simulink model "OCT07_4_cs"  (Simulink 8.8)
settings: Solver=ode5  StartTime=0.0  StopTime=inf  FixedStep=1/20  RelTol=1e-3
model workspace (MAT data in the model file):
  mbox_table : struct (value not decoded)
  model_closed = 0
  sim_status = 0
PreLoadFcn:
  | check_NUTS_defined;
  | 
  | assignin('base',['model_closed_' bdroot],false);
InitFcn:
  | PreScanExperimentInitFcn(bdroot)
StopFcn:
  | PreScanExperimentStopFcn(bdroot)
undefined symbols (not defined in the file): DiscIntNeverNeededParam, InitImageOutputDir, lf, lr
libraries: PreScanSimulinkLibrary x4, PreScanUsefulBlocks x3
(part 1 of 2)
CloseFcn:
  | evalin('base',['clear model_closed_' bdroot]);
settings Model: Creator=PRESCAN  LastModifiedBy=yuntao891011
settings OptimizationCC: ExpressionDepthLimit=2147483647  InitFltsAndDblsToZero=on
settings DebuggingCC: SaveWithParameterizedLinksMsg=none  SignalResolutionControl=TryResolveAllWithWarning  MultiTaskDSMMsg=warning  MultiTaskCondExecSysMsg=none
settings GRTTargetCC: TargetFcnLib=ansi_tfl_tmw.mat

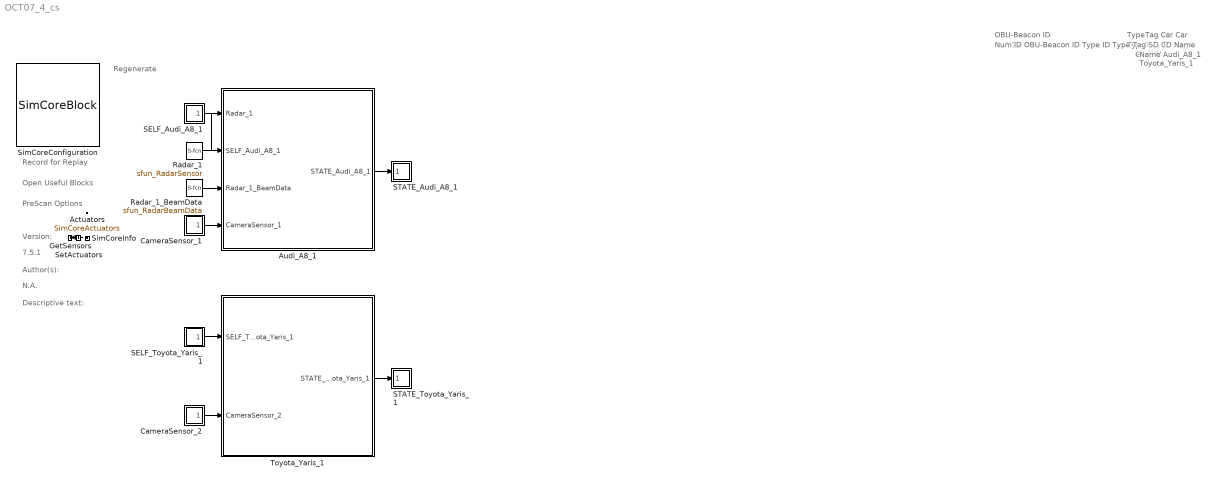
== system OCT07_4_cs ==
  note: Regenerate
  note: Record for Replay
  note: Open Useful Blocks
  note: PreScan Options
  note: Version:
  note: 7.5.1
  note: Author(s):
  note: N.A.
  note: Descriptive text:
  note: ID
      |
      | 2
      | 12
  note: OBU-Beacon ID
  note: TypeID
      |
      | 1
      | 1
  note: TypeTag
      |
      | Car
      | Car
  note: SD
      |
      | Y
      | Y
  note: CD
      |
      | N
      | N
  note: Name
      |
      | Audi_A8_1
      | Toyota_Yaris_1
  note: Num ID OBU-Beacon ID Type ID Type Tag SD CD Name
  Actuators : DataStoreMemory  DataStoreName=SimCoreActuators  InitialValue=zeros(30,1)  ShowAdditionalParam=off
  Audi_A8_1 : Subsystem  Tag=WorldObjectSubSystem  InitFcn=UniqueId = '14';
      mask Display: image(imread('Audi_A8.jpg'));color('white');text(0,0,' ID=2\n')
  CameraSensor_1 : Subsystem  Tag=CameraSensor  Priority=3  mask(PreScan Source Block: Camera Sensor){}
      mask help: The Camera Sensor provides a color or monochrome image.
      settings: DeleteFcn=PreScanBlockDeleteFcn;
      mask Help: eval('openHelp(457)')
      mask Display: image(imread('CameraSensor.png'))
  CameraSensor_2 : Subsystem  Tag=CameraSensor  Priority=3  mask(PreScan Source Block: Camera Sensor){}
      mask help: The Camera Sensor provides a color or monochrome image.
      settings: DeleteFcn=PreScanBlockDeleteFcn;
      mask Help: eval('openHelp(457)')
      mask Display: image(imread('CameraSensor.png'))
  GetSensors : Subsystem  Tag=GetSensors  Priority=2  mask(PreScan Simulation Core Block){NrOfSensors=16, TimeStep=1/20}
      mask prompts: NrOfSensors "Number of sensor values"; TimeStep "Timestep [s]"
      mask help:
      | Please do not remove this block from the PreScan compilation sheet,
      | as it contains essential configuration parameters for a PreScan simulation.
      settings: DeleteFcn=PreScanBlockDeleteFcn;
  Radar_1 : S-Function  Priority=3  LoadFcn=load('PrescanScannerSensorData.mat');load('PrescanScannerSensorMessage.mat')  FunctionName=sfun_RadarSensor  Parameters=timestepMask maxInputMessages maxOutputMessages sensorID detectableObjects  SFunctionDeploymentMode=off  EnableBusSupport=off  mask{timestepMask=1/20, maxInputMessages=0, maxOutputMessages=7, sensorID=15, detectableObjects=7}
      mask prompts: timestepMask "MATLAB timestep:"; maxInputMessages "Max input messages:"; maxOutputMessages "Max output messages:"; sensorID "Sensor ID:"; detectableObjects "Max detectable objects:"
      mask help: RadarSensor I/O
      mask Display: image(imread('Radar.png'))
  Radar_1_BeamData : S-Function  Priority=3  LoadFcn=load('PrescanScannerSensorBeamData.mat');load('PrescanScannerSensorBeamMessage.mat')  FunctionName=sfun_RadarBeamData  Parameters=timestepMask maxInputMessages maxOutputMessages sensorID detectableObjects  SFunctionDeploymentMode=off  EnableBusSupport=off  mask{timestepMask=1/20, maxInputMessages=0, maxOutputMessages=1, sensorID=15, detectableObjects=1}
      mask prompts: timestepMask "MATLAB timestep:"; maxInputMessages "Max input messages:"; maxOutputMessages "Max output messages:"; sensorID "Sensor ID:"; detectableObjects "Max detectable objects:"
      mask help: RadarSensor I/O
      mask Display: image(imread('BeamInfo.png'))
  SELF_Audi_A8_1 : Subsystem  Tag=SELF  Priority=3  mask(PreScan Source Block: SELF){PortName=SELF_Audi_A8_1, PortIndex=0, PortWidth=8, TimeStep=1/20}
      mask prompts: PortName "Auto-Assigned: Port Name [-]"; PortIndex "Auto-Assigned: Port Index [-]"; PortWidth "Auto-Assigned: Port Dimensions"; TimeStep "Auto-Assigned: Upload Period [s]"
      mask help:
      | The SELF port shows (state) information of the actor itself. The outputs are position in the experiment's axis system and the GPS coordinates, and the object's absolute velocity and compass heading.
      |
      | For more information, please click Help.
      settings: DeleteFcn=PreScanBlockDeleteFcn;
      mask Help: eval('openHelp(462)')
      mask Display: image(imread('GPS.png'))
  SELF_Toyota_Yaris_1 : Subsystem  Tag=SELF  Priority=3  mask(PreScan Source Block: SELF){PortName=SELF_Toyota_Yaris_1, PortIndex=8, PortWidth=8, TimeStep=1/20}
      mask prompts: PortName "Auto-Assigned: Port Name [-]"; PortIndex "Auto-Assigned: Port Index [-]"; PortWidth "Auto-Assigned: Port Dimensions"; TimeStep "Auto-Assigned: Upload Period [s]"
      mask help:
      | The SELF port shows (state) information of the actor itself. The outputs are position in the experiment's axis system and the GPS coordinates, and the object's absolute velocity and compass heading.
      |
      | For more information, please click Help.
      settings: DeleteFcn=PreScanBlockDeleteFcn;
      mask Help: eval('openHelp(462)')
      mask Display: image(imread('GPS.png'))
  STATE_Audi_A8_1 : Subsystem  Tag=State  Priority=0  mask(PreScan Sink Block: State){x0=0.70359420776367188, y0=-3.0454330444335937, z0=0.55, Roll0=0, Pitch0=0, Yaw0=0, TimeStep=1/20}
      mask prompts: x0 "Ini x-position VEHICLE wrt GLOBAL axis system [m]"; y0 "Ini y-position VEHICLE wrt GLOBAL axis system [m]"; z0 "Ini z-position VEHICLE wrt GLOBAL axis system [m]"; Roll0 "Ini roll-angle BODY wrt VEHICLE axis system [deg]"; Pitch0 "Ini pitch-angle BODY wrt VEHICLE axis system [deg]"; Yaw0 "Ini yaw-angle VEHICLE wrt GLOBAL axis system [deg]"; TimeStep "Time Step [s]"
      mask help:
      | The Actor State contains a vector signal of size (9x1), containing the following signals:
      |
      | -  Position                  (x,y,z)                                     [m]
      | -  Velocity                  (vx,vy,vz)                               [m/s]
      | -  Angles                    (Roll, Pitch, Yaw)                   [rad]
      |
      | The Actor state is defined in the global axis system.
      | The state is superponed on the Initial position defined in the GUI.
      |
      | For more information, please click Help.
      settings: DeleteFcn=PreScanBlockDeleteFcn;
      mask Help: eval('openHelp(222)')
      mask Display: image(imread('State.png'))
  STATE_Toyota_Yaris_1 : Subsystem  Tag=State  Priority=0  mask(PreScan Sink Block: State){x0=-12.185623168945313, y0=-3.0852584838867187, z0=0.57, Roll0=0, Pitch0=0, Yaw0=0, TimeStep=1/20}
      mask prompts: x0 "Ini x-position VEHICLE wrt GLOBAL axis system [m]"; y0 "Ini y-position VEHICLE wrt GLOBAL axis system [m]"; z0 "Ini z-position VEHICLE wrt GLOBAL axis system [m]"; Roll0 "Ini roll-angle BODY wrt VEHICLE axis system [deg]"; Pitch0 "Ini pitch-angle BODY wrt VEHICLE axis system [deg]"; Yaw0 "Ini yaw-angle VEHICLE wrt GLOBAL axis system [deg]"; TimeStep "Time Step [s]"
      mask help:
      | The Actor State contains a vector signal of size (9x1), containing the following signals:
      |
      | -  Position                  (x,y,z)                                     [m]
      | -  Velocity                  (vx,vy,vz)                               [m/s]
      | -  Angles                    (Roll, Pitch, Yaw)                   [rad]
      |
      | The Actor state is defined in the global axis system.
      | The state is superponed on the Initial position defined in the GUI.
      |
      | For more information, please click Help.
      settings: DeleteFcn=PreScanBlockDeleteFcn;
      mask Help: eval('openHelp(222)')
      mask Display: image(imread('State.png'))
  SetActuators : Subsystem  Tag=SetActuators  Priority=1  mask(PreScan Simulation Core Block){TimeStep=1/20, NrOfActuators=30}
      mask prompts: TimeStep "Timestep [s]"; NrOfActuators "Number of actuator values"
      mask help:
      | Please do not remove this block from the PreScan compilation sheet,
      | as it contains essential configuration parameters for a PreScan simulation.
      settings: DeleteFcn=PreScanBlockDeleteFcn;
  SimCoreConfiguration : M-S-Function  Tag=SimCoreConfiguration  Description=AFF8662A0A05274BB8B75CAA8617EE4EF722880921021BB04CFBF9D9D8032257  FunctionName=SimCoreBlock  Parameters=ExperimentXML PortsXML SimulationCore HostName CheckStart EnableLog RfR EnableGPUAccel ShowComputationTime  mask(PreScan Simulation Core Configurator){SimulationCore=NUTS, HostName=0, CheckStart=0, prescanversion='7.5.1', EnableLog=off, RfR=0, EnableGPUAccel=off, ShowComputationTime=off}
      mask prompts: SimulationCore "Simulation Core"; HostName "Simulation Host"; CheckStart "Show START Dialog"; prescanversion "PreScan Version"; EnableLog "Create TA Log"; RfR "Record for Replay"; EnableGPUAccel "Enable GPU Acceleration"; ShowComputationTime "Show ComputationTime Scope"
      mask help:
      | Please do not remove this block from the PreScan compilation sheet,
      | as it contains essential configuration parameter for a PreScan simulation.
      mask init:
      | model = bdroot;
      | ExperimentXML = [model(1:end-3) '.pex'];
      | PortsXML = [model '_ports.pcd'];
      settings: DeleteFcn=PreScanBlockDeleteFcn;  ModelCloseFcn=assignin('base',['model_closed_' bdroot],true);
      mask Help: eval('openHelp(812)')
      mask Display: image(imread('prescanlogo.ico'))
  SimCoreInfo : Subsystem  Tag=SimCoreInfo
  Toyota_Yaris_1 : Subsystem  Tag=WorldObjectSubSystem  InitFcn=UniqueId = '28';
      mask Display: image(imread('Toyota_Yaris.jpg'));color('white');text(0,0,' ID=12\n')
  wires:
  SetActuators/1(dummy) -> GetSensors/1(dummy)
  Audi_A8_1/1(STATE_Audi_A8_1) -> STATE_Audi_A8_1/1(State)
  SELF_Audi_A8_1/1(U) -> Audi_A8_1/2(SELF_Audi_A8_1)
  Radar_1/1 -> Audi_A8_1/1(Radar_1)
  Radar_1_BeamData/1 -> Audi_A8_1/3(Radar_1_BeamData)
  CameraSensor_1/1(U1) -> Audi_A8_1/4(CameraSensor_1)
  Toyota_Yaris_1/1(STATE_Toyota_Yaris_1) -> STATE_Toyota_Yaris_1/1(State)
  SELF_Toyota_Yaris_1/1(U) -> Toyota_Yaris_1/1(SELF_Toyota_Yaris_1)
  CameraSensor_2/1(U1) -> Toyota_Yaris_1/2(CameraSensor_2)

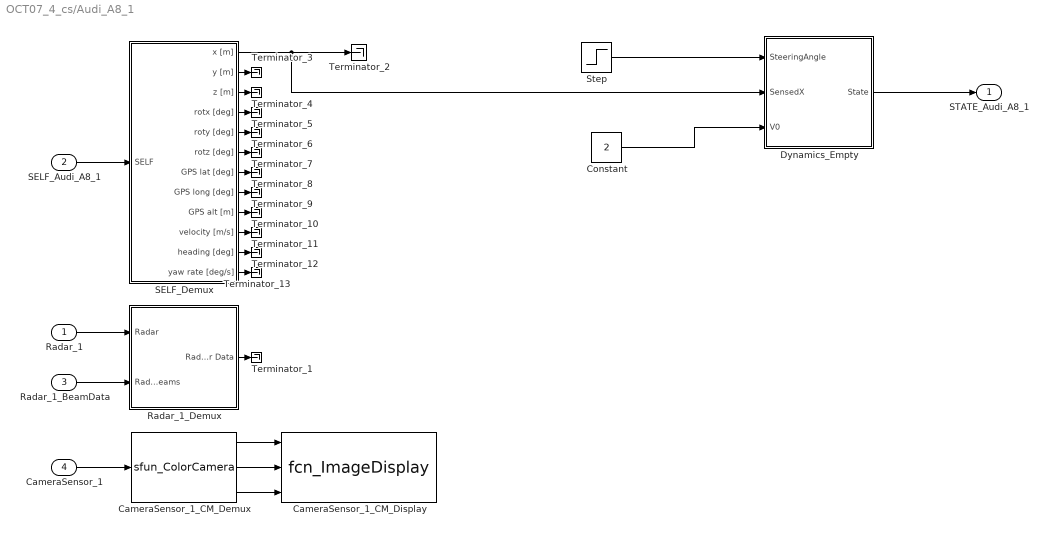
== system OCT07_4_cs/Audi_A8_1 ==
  Radar_1 : Inport  Tag=RadarInport  OutDataTypeStr=Bus: PRESCAN_SCANNERSENSORMESSAGE
  SELF_Audi_A8_1 : Inport  Tag=SELFInport  Port=2
  Radar_1_BeamData : Inport  Tag=RadarInport  Port=3  OutDataTypeStr=Bus: PRESCAN_SCANNERSENSORBEAMMESSAGE
  CameraSensor_1 : Inport  Tag=CameraSensorInport  Port=4  SampleTime=1/20
  CameraSensor_1_CM_Demux : S-Function  Tag=CameraSensor_Color_Demux  FunctionName=sfun_ColorCamera  Parameters=[VerticalResolution HorizontalResolution] FrameRate SensorName CameraType SharedMemTag SharedMemRightTag DataType  SFunctionDeploymentMode=off  EnableBusSupport=off  mask{HorizontalResolution=320, VerticalResolution=240, FrameRate=20, SensorName=CameraSensor_1, CameraType=Mono, SharedMemTag=CameraSensor_1_monoBeam_viewer_RGB, SharedMemRightTag=CameraSensor_1_StereoRight_viewer_RGB, DataType=uint8}
      mask prompts: HorizontalResolution "User Specified: Horizontal Resolution [pixels]"; VerticalResolution "User Specified: Vertical Resolution [pixels]"; FrameRate "User Specified: Frame Rate [Hz]"; SensorName "User Specified: Camera Sensor Name"; CameraType "Camera Type"; SharedMemTag "Tag for shared memory for main img"; SharedMemRightTag "Tag for shared memory for right img"; DataType "Image Data Type"
      mask init:
      | if CameraType==1
      |     CameraTypeName='MONO';
      |     PortNumber=0;
      | else
      |     CameraTypeName='STEREO';
      |     PortNumber=3;
      | end
      settings: DeleteFcn=PreScanBlockDeleteFcn;
      mask TypeOptions CameraType: Mono | Stereo
      mask TypeOptions DataType: uint8 | single
      mask Display:
      | fprintf('%s CAMERA:\n Color\n %s \n V: %d x %d \n %d fps',CameraTypeName,SensorName,VerticalResolution,HorizontalResolution,FrameRate)
      | port_label('output',1,'R')
      | port_label('output',2,'G')
      | port_label('output',3,'B')
      | port_label('output',PortNumber+1,'R')
      | port_label('output',PortNumber+2,'G')
      | port_label('output',PortNumber+3,'B')
  CameraSensor_1_CM_Display : M-S-Function  Tag=CameraSensor_Color_Display  InitFcn=InitImageOutputDir(gcb);  FunctionName=fcn_ImageDisplay  Parameters=SensorName EnableDisplay EnablePosition DisplayPosition FigureHandle SaveResults BitmapFormat TempOutputDir CameraType DataType  mask(PreScan Color Display Block){SensorName=CameraSensor_1, EnableDisplay=on, EnablePosition=off, DisplayPosition=[10 10 320 240], FigureHandle=200, SaveResults=off, Format=PNG, TempOutputDir=0, CameraType=Mono, DataType=uint8}
      mask prompts: SensorName "User Specified: Title of Display"; EnableDisplay "Active"; EnablePosition "Set Display window position"; DisplayPosition "Display window position [xpos ypos width height]"; FigureHandle "Unique Handle"; SaveResults "Save results"; TempOutputDir "OutputDir"; CameraType "Camera Type"; DataType "Image Data Type"
      mask help: This block displays the RGB output of a PreScan camera sensor.
      mask init:
      | if EnableDisplay
      |     EnableString='';
      |     EnableColor='gray';
      | else
      |     EnableString='INACTIVE';
      |     EnableColor='red';
      | end
      | switch Format
      |     case 1
      |         BitmapFormat = 'png';
      |     case 2
      |         BitmapFormat = 'bmp';
      |     case 3
      |         BitmapFormat = 'jpg';
      | end 
      | if CameraType==1
      |     CameraTypeName='MONO';
      |     PortNumber=0;
      | else
      |     CameraTypeName='STEREO';
      |     PortNumber=3;
      | end
      settings: CopyFcn=CopyFcnDisplay  DeleteFcn=PreScanBlockDeleteFcn;  ModelCloseFcn=fcn_ImageDisplay_ModelCloseFcn
      mask Help: eval('openHelp(457)')
      mask Callback EnablePosition:
      | MV=get_param(gcb,'MaskVisibilities');
      | if strcmp(get_param(gcb,'EnablePosition'),'on')
      |     MV{4}='on';
      | else
      |     MV{4}='off';
      | end
      | set_param(gcb,'MaskVisibilities',MV);
      mask TypeOptions Format: PNG | BMP | JPG
      mask TypeOptions CameraType: Mono | Stereo
      mask TypeOptions DataType: uint8 | single
      mask Display:
      | color(EnableColor);
      | fprintf('%s\n DISPLAY:\n Color \n %s',EnableString,SensorName)
      | port_label('input',1,'R')
      | port_label('input',2,'G')
      | port_label('input',3,'B')
      | port_label('input',PortNumber+1,'R')
      | port_label('input',PortNumber+2,'G')
      | port_label('input',PortNumber+3,'B')
  Constant : Constant  Value=2
  Dynamics_Empty : Subsystem  Tag=Dynamics_Empty
  Radar_1_Demux : Subsystem  TreatAsAtomicUnit=on  mask(PreScan Demux Block: Radar){MAXMESSAGES=7}
      mask prompts: MAXMESSAGES "Number of Objects"
      mask help:
      | The Radar Sensor is a detailed sensor based on a physical radar
      | model that includes Antenna GAIN Maps (AGM) and atmospheric
      | attenuation.
      |
      | For more information, please click Help.
      mask Help: eval('openHelp(431)')
      mask Display:
      | port_label('input',1,'Radar')
      | port_label('output',1,'Radar Data')
  SELF_Demux : Subsystem  Tag=DemuxSELF  mask(PreScan Demux Block:){}
      settings: DeleteFcn=PreScanBlockDeleteFcn;
      mask Display:
      | port_label('output',1,'x [m]')
      | port_label('output',2,'y [m]')
      | port_label('output',3,'z [m]','texmode','on')
      | port_label('output',4,'Rotx [deg]','texmode','on')
      | port_label('output',5,'Roty [deg]','texmode','on')
      | port_label('output',6,'Rotz [deg]','texmode','on')
      | port_label('output',7,'GPS lat [deg]','texmode','on')
      | port_label('output',8,'GPS long [deg]','texmode','on')
      | port_label('output',9,'GPS alt [m]','texmode','on')
      | port_label('output',10,'Velocity [m/s]')
      | port_label('output',11,'Heading [deg]')
      | port_label('output',12,'Yaw rate [deg/s]')
  Step : Step  Time=0  After=10  SampleTime=0
  Terminator_{1..13} (13 alike) : Terminator
  STATE_Audi_A8_1 : Outport  Tag=StateOutport
  wires:
  Step/1 -> Dynamics_Empty/1(SteeringAngle)
  Constant/1 -> Dynamics_Empty/3(V0)
  SELF_Audi_A8_1/1 -> SELF_Demux/1(SELF)
  Radar_1/1 -> Radar_1_Demux/1(Radar)
  Radar_1_BeamData/1 -> Radar_1_Demux/2(RadarBeams)
  CameraSensor_1_CM_Demux/1 -> CameraSensor_1_CM_Display/1
  CameraSensor_1_CM_Demux/2 -> CameraSensor_1_CM_Display/2
  CameraSensor_1_CM_Demux/3 -> CameraSensor_1_CM_Display/3
  CameraSensor_1/1 -> CameraSensor_1_CM_Demux/1
  Dynamics_Empty/1(State) -> STATE_Audi_A8_1/1
  Radar_1_Demux/1(Radar Data) -> Terminator_1/1
  SELF_Demux/1(x [m]) -> Dynamics_Empty/2("SensedX "), Terminator_2/1
  SELF_Demux/2(y [m]) -> Terminator_3/1
  SELF_Demux/3(z [m]) -> Terminator_4/1
  SELF_Demux/4(rotx [deg]) -> Terminator_5/1
  SELF_Demux/5(roty [deg]) -> Terminator_6/1
  SELF_Demux/6(rotz [deg]) -> Terminator_7/1
  SELF_Demux/7(GPS lat [deg]) -> Terminator_8/1
  SELF_Demux/8(GPS long [deg]) -> Terminator_9/1
  SELF_Demux/9(GPS alt [m]) -> Terminator_10/1
  SELF_Demux/10(velocity [m/s]) -> Terminator_11/1
  SELF_Demux/11(heading [deg]) -> Terminator_12/1
  SELF_Demux/12(yaw rate [deg/s]) -> Terminator_13/1

== system OCT07_4_cs/CameraSensor_1 ==
  Demux : Demux  Outputs=[1 -1]
  Terminator : Terminator
  U1 : Outport
  wires:
  Demux/2 -> Terminator/1
  Demux/1 -> U1/1
  [SimCoreSensors] -> Demux/1

== system OCT07_4_cs/CameraSensor_2 ==
  Demux : Demux  Outputs=[1 -1]
  Terminator : Terminator
  U1 : Outport
  wires:
  Demux/2 -> Terminator/1
  Demux/1 -> U1/1
  [SimCoreSensors] -> Demux/1

== system OCT07_4_cs/GetSensors ==
  dummy : Inport
  GetSensors : M-S-Function  FunctionName=GetSensorsBlock  Parameters=TimeStep NrOfSensors
  tag scope: SimCoreSensors=global
  wires:
  GetSensors/1 -> [SimCoreSensors]
  dummy/1 -> GetSensors/1

== system OCT07_4_cs/SELF_Audi_A8_1 ==
  Selector : Selector  IndexMode=Zero-based  IndexOptions=Starting index (dialog)  Indices=PortIndex  OutputSizes=PortWidth(1)
  U : Outport
  wires:
  Selector/1 -> U/1
  [SimCoreSensors] -> Selector/1

== system OCT07_4_cs/SELF_Toyota_Yaris_1 ==
  Selector : Selector  IndexMode=Zero-based  IndexOptions=Starting index (dialog)  Indices=PortIndex  OutputSizes=PortWidth(1)
  U : Outport
  wires:
  Selector/1 -> U/1
  [SimCoreSensors] -> Selector/1

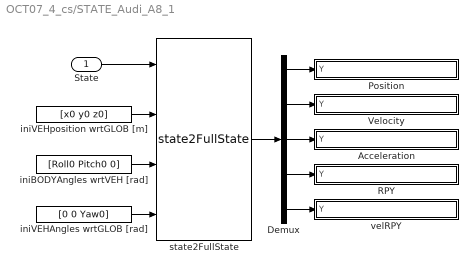
== system OCT07_4_cs/STATE_Audi_A8_1 ==
  State : Inport  SampleTime=TimeStep
  Acceleration : Subsystem  mask(ToSensorWorld){PortName=Acceleration_Audi_A8_1, PortIndex=6, PortWidth=3, TimeStep=1/20}
      mask prompts: PortName "Port Name [-]"; PortIndex "Index [-]"; PortWidth "Port Dimensions [-]"; TimeStep "Upload Period [s]"
      mask help: Sends signal(s) from Simulink to the Sensor World
      mask Help:
      | Sends signal(s) from Simulink to the Sensor World.
      | 
      | - Port Name [-]: specifies the name of the output terminal of the Simulink block.
      | - Index [-]: specifies the start position in the output vector sent to the Sensor World
      | - Port dimensions [-]: specifies the width (number of scalars) of the output port
      | - Upload period [s]: specifies the upload period (in seconds) of the port.
      mask Display: port_label('input', 1, PortName)
  Demux : Demux  Outputs=5
  Position : Subsystem  mask(ToSensorWorld){PortName=Position_Audi_A8_1, PortIndex=0, PortWidth=3, TimeStep=1/20}
      mask prompts: PortName "Port Name [-]"; PortIndex "Index [-]"; PortWidth "Port Dimensions [-]"; TimeStep "Upload Period [s]"
      mask help: Sends signal(s) from Simulink to the Sensor World
      mask Help:
      | Sends signal(s) from Simulink to the Sensor World.
      | 
      | - Port Name [-]: specifies the name of the output terminal of the Simulink block.
      | - Index [-]: specifies the start position in the output vector sent to the Sensor World
      | - Port dimensions [-]: specifies the width (number of scalars) of the output port
      | - Upload period [s]: specifies the upload period (in seconds) of the port.
      mask Display: port_label('input', 1, PortName)
  RPY : Subsystem  mask(ToSensorWorld){PortName=RPY_Audi_A8_1, PortIndex=9, PortWidth=3, TimeStep=1/20}
      mask prompts: PortName "Port Name [-]"; PortIndex "Index [-]"; PortWidth "Port Dimensions [-]"; TimeStep "Upload Period [s]"
      mask help: Sends signal(s) from Simulink to the Sensor World
      mask Help:
      | Sends signal(s) from Simulink to the Sensor World.
      | 
      | - Port Name [-]: specifies the name of the output terminal of the Simulink block.
      | - Index [-]: specifies the start position in the output vector sent to the Sensor World
      | - Port dimensions [-]: specifies the width (number of scalars) of the output port
      | - Upload period [s]: specifies the upload period (in seconds) of the port.
      mask Display: port_label('input', 1, PortName)
  Velocity : Subsystem  mask(ToSensorWorld){PortName=Velocity_Audi_A8_1, PortIndex=3, PortWidth=3, TimeStep=1/20}
      mask prompts: PortName "Port Name [-]"; PortIndex "Index [-]"; PortWidth "Port Dimensions [-]"; TimeStep "Upload Period [s]"
      mask help: Sends signal(s) from Simulink to the Sensor World
      mask Help:
      | Sends signal(s) from Simulink to the Sensor World.
      | 
      | - Port Name [-]: specifies the name of the output terminal of the Simulink block.
      | - Index [-]: specifies the start position in the output vector sent to the Sensor World
      | - Port dimensions [-]: specifies the width (number of scalars) of the output port
      | - Upload period [s]: specifies the upload period (in seconds) of the port.
      mask Display: port_label('input', 1, PortName)
  iniBODYAngles wrtVEH [rad] : Constant  Value=[Roll0 Pitch0 0]  SampleTime=TimeStep
  iniVEHAngles wrtGLOB [rad] : Constant  Value=[0 0 Yaw0]  SampleTime=TimeStep
  iniVEHposition wrtGLOB [m] : Constant  Value=[x0 y0 z0]  SampleTime=TimeStep
  state2FullState : PreScanSimulinkLibrary/state2FullState  SystemSampleTime=-1
  velRPY : Subsystem  mask(ToSensorWorld){PortName=velRPY_Audi_A8_1, PortIndex=12, PortWidth=3, TimeStep=1/20}
      mask prompts: PortName "Port Name [-]"; PortIndex "Index [-]"; PortWidth "Port Dimensions [-]"; TimeStep "Upload Period [s]"
      mask help: Sends signal(s) from Simulink to the Sensor World
      mask Help:
      | Sends signal(s) from Simulink to the Sensor World.
      | 
      | - Port Name [-]: specifies the name of the output terminal of the Simulink block.
      | - Index [-]: specifies the start position in the output vector sent to the Sensor World
      | - Port dimensions [-]: specifies the width (number of scalars) of the output port
      | - Upload period [s]: specifies the upload period (in seconds) of the port.
      mask Display: port_label('input', 1, PortName)
  wires:
  Demux/5 -> velRPY/1(Y)
  Demux/4 -> RPY/1(Y)
  Demux/3 -> Acceleration/1(Y)
  Demux/2 -> Velocity/1(Y)
  Demux/1 -> Position/1(Y)
  State/1 -> state2FullState/1
  state2FullState/1 -> Demux/1
  iniVEHposition wrtGLOB [m]/1 -> state2FullState/2
  iniBODYAngles wrtVEH [rad]/1 -> state2FullState/3
  iniVEHAngles wrtGLOB [rad]/1 -> state2FullState/4

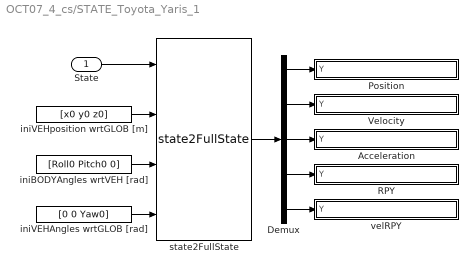
== system OCT07_4_cs/STATE_Toyota_Yaris_1 ==
  State : Inport  SampleTime=TimeStep
  Acceleration : Subsystem  mask(ToSensorWorld){PortName=Acceleration_Toyota_Yaris_1, PortIndex=21, PortWidth=3, TimeStep=1/20}
      mask prompts: PortName "Port Name [-]"; PortIndex "Index [-]"; PortWidth "Port Dimensions [-]"; TimeStep "Upload Period [s]"
      mask help: Sends signal(s) from Simulink to the Sensor World
      mask Help:
      | Sends signal(s) from Simulink to the Sensor World.
      | 
      | - Port Name [-]: specifies the name of the output terminal of the Simulink block.
      | - Index [-]: specifies the start position in the output vector sent to the Sensor World
      | - Port dimensions [-]: specifies the width (number of scalars) of the output port
      | - Upload period [s]: specifies the upload period (in seconds) of the port.
      mask Display: port_label('input', 1, PortName)
  Demux : Demux  Outputs=5
  Position : Subsystem  mask(ToSensorWorld){PortName=Position_Toyota_Yaris_1, PortIndex=15, PortWidth=3, TimeStep=1/20}
      mask prompts: PortName "Port Name [-]"; PortIndex "Index [-]"; PortWidth "Port Dimensions [-]"; TimeStep "Upload Period [s]"
      mask help: Sends signal(s) from Simulink to the Sensor World
      mask Help:
      | Sends signal(s) from Simulink to the Sensor World.
      | 
      | - Port Name [-]: specifies the name of the output terminal of the Simulink block.
      | - Index [-]: specifies the start position in the output vector sent to the Sensor World
      | - Port dimensions [-]: specifies the width (number of scalars) of the output port
      | - Upload period [s]: specifies the upload period (in seconds) of the port.
      mask Display: port_label('input', 1, PortName)
  RPY : Subsystem  mask(ToSensorWorld){PortName=RPY_Toyota_Yaris_1, PortIndex=24, PortWidth=3, TimeStep=1/20}
      mask prompts: PortName "Port Name [-]"; PortIndex "Index [-]"; PortWidth "Port Dimensions [-]"; TimeStep "Upload Period [s]"
      mask help: Sends signal(s) from Simulink to the Sensor World
      mask Help:
      | Sends signal(s) from Simulink to the Sensor World.
      | 
      | - Port Name [-]: specifies the name of the output terminal of the Simulink block.
      | - Index [-]: specifies the start position in the output vector sent to the Sensor World
      | - Port dimensions [-]: specifies the width (number of scalars) of the output port
      | - Upload period [s]: specifies the upload period (in seconds) of the port.
      mask Display: port_label('input', 1, PortName)
  Velocity : Subsystem  mask(ToSensorWorld){PortName=Velocity_Toyota_Yaris_1, PortIndex=18, PortWidth=3, TimeStep=1/20}
      mask prompts: PortName "Port Name [-]"; PortIndex "Index [-]"; PortWidth "Port Dimensions [-]"; TimeStep "Upload Period [s]"
      mask help: Sends signal(s) from Simulink to the Sensor World
      mask Help:
      | Sends signal(s) from Simulink to the Sensor World.
      | 
      | - Port Name [-]: specifies the name of the output terminal of the Simulink block.
      | - Index [-]: specifies the start position in the output vector sent to the Sensor World
      | - Port dimensions [-]: specifies the width (number of scalars) of the output port
      | - Upload period [s]: specifies the upload period (in seconds) of the port.
      mask Display: port_label('input', 1, PortName)
  iniBODYAngles wrtVEH [rad] : Constant  Value=[Roll0 Pitch0 0]  SampleTime=TimeStep
  iniVEHAngles wrtGLOB [rad] : Constant  Value=[0 0 Yaw0]  SampleTime=TimeStep
  iniVEHposition wrtGLOB [m] : Constant  Value=[x0 y0 z0]  SampleTime=TimeStep
  state2FullState : PreScanSimulinkLibrary/state2FullState  SystemSampleTime=-1
  velRPY : Subsystem  mask(ToSensorWorld){PortName=velRPY_Toyota_Yaris_1, PortIndex=27, PortWidth=3, TimeStep=1/20}
      mask prompts: PortName "Port Name [-]"; PortIndex "Index [-]"; PortWidth "Port Dimensions [-]"; TimeStep "Upload Period [s]"
      mask help: Sends signal(s) from Simulink to the Sensor World
      mask Help:
      | Sends signal(s) from Simulink to the Sensor World.
      | 
      | - Port Name [-]: specifies the name of the output terminal of the Simulink block.
      | - Index [-]: specifies the start position in the output vector sent to the Sensor World
      | - Port dimensions [-]: specifies the width (number of scalars) of the output port
      | - Upload period [s]: specifies the upload period (in seconds) of the port.
      mask Display: port_label('input', 1, PortName)
  wires:
  Demux/5 -> velRPY/1(Y)
  Demux/4 -> RPY/1(Y)
  Demux/3 -> Acceleration/1(Y)
  Demux/2 -> Velocity/1(Y)
  Demux/1 -> Position/1(Y)
  State/1 -> state2FullState/1
  state2FullState/1 -> Demux/1
  iniVEHposition wrtGLOB [m]/1 -> state2FullState/2
  iniBODYAngles wrtVEH [rad]/1 -> state2FullState/3
  iniVEHAngles wrtGLOB [rad]/1 -> state2FullState/4

== system OCT07_4_cs/SetActuators ==
  Bus Creator : BusCreator  Inputs=1
  Data Store Read : DataStoreRead  DataStoreName=SimCoreActuators  SampleTime=TimeStep
  SendActuators : M-S-Function  FunctionName=SendActuatorsBlock  Parameters=TimeStep NrOfActuators
  dummy : Outport
  tag scope: SimCoreInfo=global
  wires:
  Bus Creator/1 -> [SimCoreInfo]  "SimCore"
  SendActuators/2 -> Bus Creator/1  "ComputationTime[s]"
  SendActuators/1 -> dummy/1
  Data Store Read/1 -> SendActuators/1

== system OCT07_4_cs/SimCoreInfo ==
  Bus Selector : BusSelector  OutputSignals=ComputationTime[s]
  Time : Scope
  wires:
  Bus Selector/1 -> Time/1  "<ComputationTime[s]>"
  [SimCoreInfo] -> Bus Selector/1

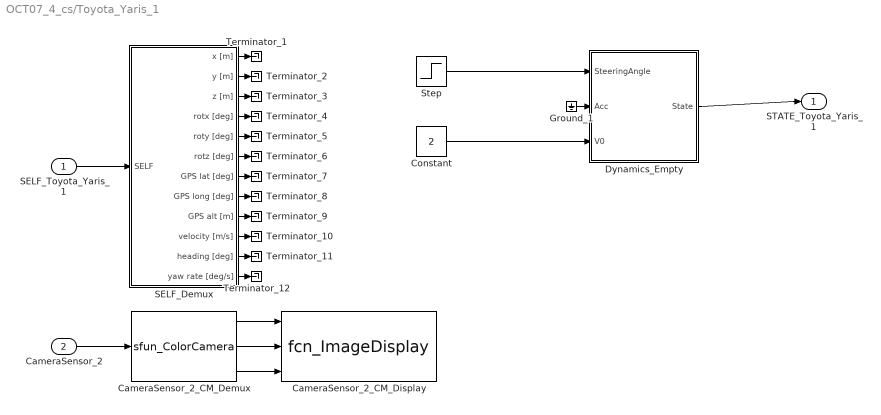
== system OCT07_4_cs/Toyota_Yaris_1 ==
  SELF_Toyota_Yaris_1 : Inport  Tag=SELFInport
  CameraSensor_2 : Inport  Tag=CameraSensorInport  Port=2  SampleTime=1/20
  CameraSensor_2_CM_Demux : S-Function  Tag=CameraSensor_Color_Demux  FunctionName=sfun_ColorCamera  Parameters=[VerticalResolution HorizontalResolution] FrameRate SensorName CameraType SharedMemTag SharedMemRightTag DataType  SFunctionDeploymentMode=off  EnableBusSupport=off  mask{HorizontalResolution=500, VerticalResolution=375, FrameRate=20, SensorName=CameraSensor_2, CameraType=Mono, SharedMemTag=CameraSensor_2_monoBeam_viewer_RGB, SharedMemRightTag=CameraSensor_2_StereoRight_viewer_RGB, DataType=uint8}
      mask prompts: HorizontalResolution "User Specified: Horizontal Resolution [pixels]"; VerticalResolution "User Specified: Vertical Resolution [pixels]"; FrameRate "User Specified: Frame Rate [Hz]"; SensorName "User Specified: Camera Sensor Name"; CameraType "Camera Type"; SharedMemTag "Tag for shared memory for main img"; SharedMemRightTag "Tag for shared memory for right img"; DataType "Image Data Type"
      mask init:
      | if CameraType==1
      |     CameraTypeName='MONO';
      |     PortNumber=0;
      | else
      |     CameraTypeName='STEREO';
      |     PortNumber=3;
      | end
      settings: DeleteFcn=PreScanBlockDeleteFcn;
      mask TypeOptions CameraType: Mono | Stereo
      mask TypeOptions DataType: uint8 | single
      mask Display:
      | fprintf('%s CAMERA:\n Color\n %s \n V: %d x %d \n %d fps',CameraTypeName,SensorName,VerticalResolution,HorizontalResolution,FrameRate)
      | port_label('output',1,'R')
      | port_label('output',2,'G')
      | port_label('output',3,'B')
      | port_label('output',PortNumber+1,'R')
      | port_label('output',PortNumber+2,'G')
      | port_label('output',PortNumber+3,'B')
  CameraSensor_2_CM_Display : M-S-Function  Tag=CameraSensor_Color_Display  InitFcn=InitImageOutputDir(gcb);  FunctionName=fcn_ImageDisplay  Parameters=SensorName EnableDisplay EnablePosition DisplayPosition FigureHandle SaveResults BitmapFormat TempOutputDir CameraType DataType  mask(PreScan Color Display Block){SensorName=CameraSensor_2, EnableDisplay=on, EnablePosition=off, DisplayPosition=[10 10 500 375], FigureHandle=1200, SaveResults=off, Format=PNG, TempOutputDir=0, CameraType=Mono, DataType=uint8}
      mask prompts: SensorName "User Specified: Title of Display"; EnableDisplay "Active"; EnablePosition "Set Display window position"; DisplayPosition "Display window position [xpos ypos width height]"; FigureHandle "Unique Handle"; SaveResults "Save results"; TempOutputDir "OutputDir"; CameraType "Camera Type"; DataType "Image Data Type"
      mask help: This block displays the RGB output of a PreScan camera sensor.
      mask init: same as OCT07_4_cs/Audi_A8_1/CameraSensor_1_CM_Display
      settings: CopyFcn=CopyFcnDisplay  DeleteFcn=PreScanBlockDeleteFcn;  ModelCloseFcn=fcn_ImageDisplay_ModelCloseFcn
      mask Help: eval('openHelp(457)')
      mask Callback EnablePosition:
      | MV=get_param(gcb,'MaskVisibilities');
      | if strcmp(get_param(gcb,'EnablePosition'),'on')
      |     MV{4}='on';
      | else
      |     MV{4}='off';
      | end
      | set_param(gcb,'MaskVisibilities',MV);
      mask TypeOptions Format: PNG | BMP | JPG
      mask TypeOptions CameraType: Mono | Stereo
      mask TypeOptions DataType: uint8 | single
      mask Display:
      | color(EnableColor);
      | fprintf('%s\n DISPLAY:\n Color \n %s',EnableString,SensorName)
      | port_label('input',1,'R')
      | port_label('input',2,'G')
      | port_label('input',3,'B')
      | port_label('input',PortNumber+1,'R')
      | port_label('input',PortNumber+2,'G')
      | port_label('input',PortNumber+3,'B')
  Constant : Constant  Value=2
  Dynamics_Empty : Subsystem  Tag=Dynamics_Empty
      mask Display: port_label('output', 1, 'State');text(0,0,' Empty\n')
  Ground_1 : Ground
  SELF_Demux : Subsystem  Tag=DemuxSELF  mask(PreScan Demux Block:){}
      settings: DeleteFcn=PreScanBlockDeleteFcn;
      mask Display:
      | port_label('output',1,'x [m]')
      | port_label('output',2,'y [m]')
      | port_label('output',3,'z [m]','texmode','on')
      | port_label('output',4,'Rotx [deg]','texmode','on')
      | port_label('output',5,'Roty [deg]','texmode','on')
      | port_label('output',6,'Rotz [deg]','texmode','on')
      | port_label('output',7,'GPS lat [deg]','texmode','on')
      | port_label('output',8,'GPS long [deg]','texmode','on')
      | port_label('output',9,'GPS alt [m]','texmode','on')
      | port_label('output',10,'Velocity [m/s]')
      | port_label('output',11,'Heading [deg]')
      | port_label('output',12,'Yaw rate [deg/s]')
  Step : Step  Time=0  After=10  SampleTime=0
  Terminator_{1..12} (12 alike) : Terminator
  STATE_Toyota_Yaris_1 : Outport  Tag=StateOutport
  wires:
  Step/1 -> Dynamics_Empty/1(SteeringAngle)
  Constant/1 -> Dynamics_Empty/3(V0)
  SELF_Toyota_Yaris_1/1 -> SELF_Demux/1(SELF)
  CameraSensor_2_CM_Demux/1 -> CameraSensor_2_CM_Display/1
  CameraSensor_2_CM_Demux/2 -> CameraSensor_2_CM_Display/2
  CameraSensor_2_CM_Demux/3 -> CameraSensor_2_CM_Display/3
  CameraSensor_2/1 -> CameraSensor_2_CM_Demux/1
  Dynamics_Empty/1(State) -> STATE_Toyota_Yaris_1/1
  Ground_1/1 -> Dynamics_Empty/2("Acc ")
  SELF_Demux/1(x [m]) -> Terminator_1/1
  SELF_Demux/2(y [m]) -> Terminator_2/1
  SELF_Demux/3(z [m]) -> Terminator_3/1
  SELF_Demux/4(rotx [deg]) -> Terminator_4/1
  SELF_Demux/5(roty [deg]) -> Terminator_5/1
  SELF_Demux/6(rotz [deg]) -> Terminator_6/1
  SELF_Demux/7(GPS lat [deg]) -> Terminator_7/1
  SELF_Demux/8(GPS long [deg]) -> Terminator_8/1
  SELF_Demux/9(GPS alt [m]) -> Terminator_9/1
  SELF_Demux/10(velocity [m/s]) -> Terminator_10/1
  SELF_Demux/11(heading [deg]) -> Terminator_11/1
  SELF_Demux/12(yaw rate [deg/s]) -> Terminator_12/1

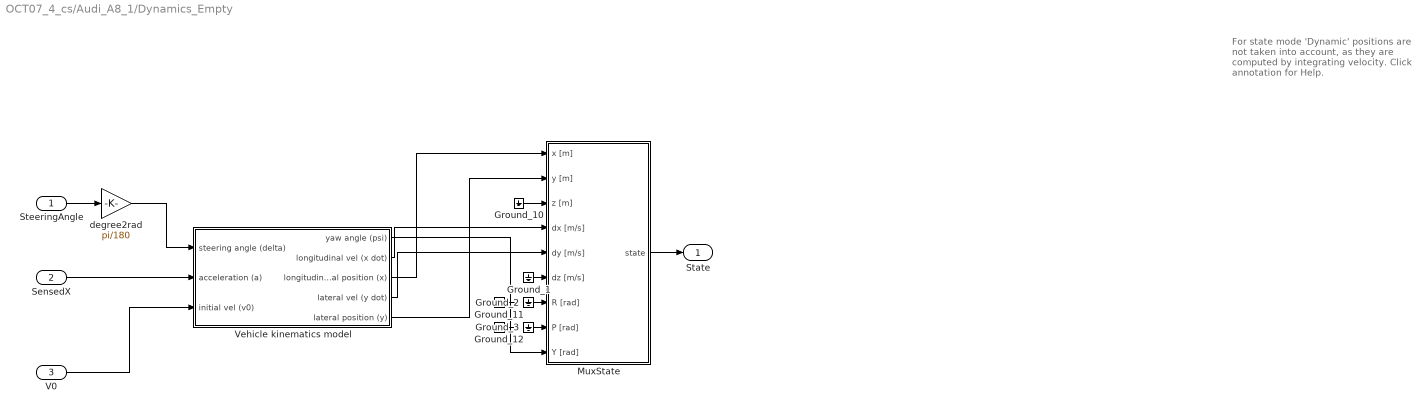
== system OCT07_4_cs/Audi_A8_1/Dynamics_Empty ==
  note: For state mode 'Dynamic' positions
      | are not taken into account, as they
      | are computed by integrating velocity.
      | Click annotation for Help.
  SteeringAngle : Inport
  "SensedX " : Inport  Port=2
  V0 : Inport  Port=3
  Ground_{1..3,10..12} (6 alike) : Ground
  MuxState : Subsystem  Tag=MuxState  mask(Empty Dynamics State Block){positioningmode=on, TimeStep=1/20}
      mask prompts: positioningmode "Positioning Mode"; TimeStep "Auto Assigned: Time Step [s]"
      mask help:
      | Build the state of an actor based on user input.
      | The user can either use positioning mode or dynamics mode.
      | - When using positioning mode the position and orientation of the actor are set directly based on the input. Expected input is relative to the initial position and orientation of the actor. It's also possible to specify the velocity of the actor, though this input isn't used, only passed on.
      | - When using dynamics mode the position input is ignored. Expected input is velocity and orientation. The velocity is relative the current orientation of the actor, while orientation is relative to its initial orientation. The position of the actor is calculated based on the velocity and orientation given.
      settings: DeleteFcn=PreScanBlockDeleteFcn;
  Vehicle kinematics model : Subsystem
  degree2rad : Gain  Gain=pi/180
  State : Outport  Tag=StateOutport
  wires:
  Vehicle kinematics model/3(longitudinal position (x)) -> MuxState/1(x [m])
  Vehicle kinematics model/5(lateral position (y)) -> MuxState/2(y [m])
  Ground_10/1 -> MuxState/3(z [m])
  Vehicle kinematics model/2(longitudinal vel (x dot)) -> MuxState/4(dx [m/s])
  Vehicle kinematics model/4(lateral vel (y dot)) -> MuxState/5(dy [m/s])
  Vehicle kinematics model/1(yaw angle (psi)) -> MuxState/9(Y [rad])
  "SensedX "/1 -> Vehicle kinematics model/2(acceleration (a))
  ? -> ?
  Ground_11/1 -> ?
  Ground_12/1 -> ?
  V0/1 -> Vehicle kinematics model/3(initial vel (v0))
  SteeringAngle/1 -> degree2rad/1
  degree2rad/1 -> Vehicle kinematics model/1(steering angle (delta))
  MuxState/1(state) -> State/1
  Ground_1/1 -> MuxState/6(dz [m/s])
  Ground_2/1 -> MuxState/7(R [rad])
  Ground_3/1 -> MuxState/8(P [rad])

== system OCT07_4_cs/Audi_A8_1/Radar_1_Demux ==
  Radar : Inport
  RadarBeams : Inport  Port=2
  Bus Creator : BusCreator  Inputs=13
  Bus Selector : BusSelector  OutputSignals=Range[m],DopplerVelocity[ms-1],DopplerVelocityX[ms-1],DopplerVelocityY[ms-1],DopplerVelocityZ[ms-1],Theta[deg],Phi[deg],TargetID[-],TargetTypeID[-],EnergyLoss[dB],Alpha[deg],Beta[deg]
  Bus Selector1 : BusSelector  OutputSignals=DATA.ActiveBeamID
  ScannerSensorLegacyBusConversion : PreScanUsefulBlocks/ScannerSensorLegacyBusConversion  MAXMESSAGES=MAXMESSAGES
  Radar Data : Outport
  wires:
  Bus Selector1/1 -> Bus Creator/1  "<ActiveBeamID>"
  RadarBeams/1 -> Bus Selector1/1
  Bus Creator/1 -> Radar Data/1
  Bus Selector/12 -> Bus Creator/13  "<Beta[deg]>"
  Bus Selector/11 -> Bus Creator/12  "<Alpha[deg]>"
  Bus Selector/10 -> Bus Creator/11  "<EnergyLoss[dB]>"
  Bus Selector/9 -> Bus Creator/10  "<TargetTypeID[-]>"
  Bus Selector/8 -> Bus Creator/9  "<TargetID[-]>"
  Bus Selector/7 -> Bus Creator/8  "<Phi[deg]>"
  Bus Selector/6 -> Bus Creator/7  "<Theta[deg]>"
  Bus Selector/5 -> Bus Creator/6  "<DopplerVelocityZ[ms-1]>"
  Bus Selector/4 -> Bus Creator/5  "<DopplerVelocityY[ms-1]>"
  Bus Selector/3 -> Bus Creator/4  "<DopplerVelocityX[ms-1]>"
  Bus Selector/2 -> Bus Creator/3  "<DopplerVelocity[ms-1]>"
  Bus Selector/1 -> Bus Creator/2  "<Range[m]>"
  ScannerSensorLegacyBusConversion/1 -> Bus Selector/1
  Radar/1 -> ScannerSensorLegacyBusConversion/1

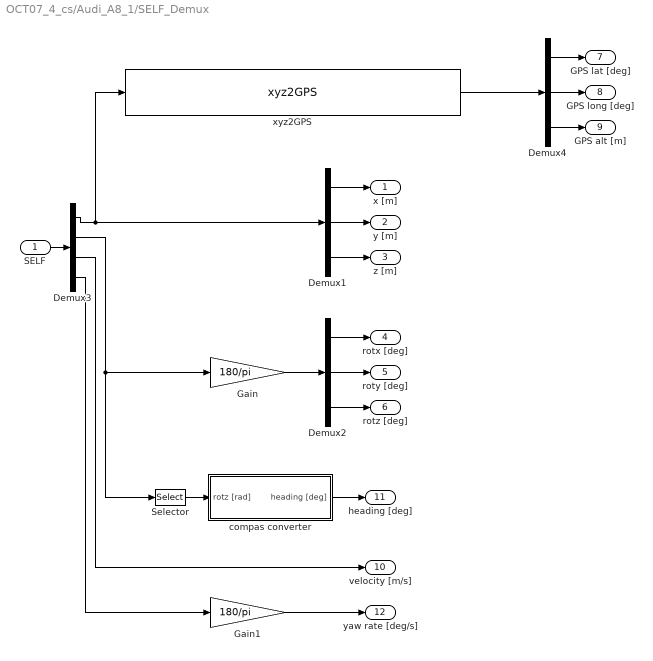
== system OCT07_4_cs/Audi_A8_1/SELF_Demux ==
  SELF : Inport
  Demux1 : Demux  Outputs=3
  Demux2 : Demux  Outputs=3
  Demux3 : Demux  Outputs=[3 3 1 1]
  Demux4 : Demux  Outputs=3
  Gain : Gain  Gain=180/pi
  Gain1 : Gain  Gain=180/pi
  Selector : Selector  InputPortWidth=3  IndexOptions=Index vector (dialog)  Indices=[3]  OutputSizes=1
  compas converter : Subsystem
  xyz2GPS : PreScanUsefulBlocks/xyz2GPS  CoordinateCount=1  GPS_base=[0.000000 0.000000 0.000]
  x [m] : Outport
  y [m] : Outport  Port=2
  z [m] : Outport  Port=3
  rotx [deg] : Outport  Port=4
  roty [deg] : Outport  Port=5
  rotz [deg] : Outport  Port=6
  GPS lat [deg] : Outport  Port=7
  GPS long [deg] : Outport  Port=8
  GPS alt [m] : Outport  Port=9
  velocity [m/s] : Outport  Port=10
  heading [deg] : Outport  Port=11
  yaw rate [deg/s] : Outport  Port=12
  wires:
  Demux3/4 -> Gain1/1
  Gain1/1 -> yaw rate [deg/s]/1
  Demux3/3 -> velocity [m/s]/1
  compas converter/1(heading [deg]) -> heading [deg]/1
  xyz2GPS/1 -> Demux4/1
  Demux4/3 -> GPS alt [m]/1
  Demux4/2 -> GPS long [deg]/1
  Demux4/1 -> GPS lat [deg]/1
  Demux3/2 -> Gain/1, Selector/1
  Demux3/1 -> xyz2GPS/1, Demux1/1
  SELF/1 -> Demux3/1
  Demux2/3 -> rotz [deg]/1
  Demux2/2 -> roty [deg]/1
  Demux2/1 -> rotx [deg]/1
  Demux1/3 -> z [m]/1
  Demux1/2 -> y [m]/1
  Demux1/1 -> x [m]/1
  Gain/1 -> Demux2/1
  Selector/1 -> compas converter/1(rotz [rad])

== system OCT07_4_cs/STATE_Audi_A8_1/Acceleration ==
  Y : Inport
  Assignment : Assignment  IndexMode=Zero-based  SampleTime=TimeStep  IndexOptions=Starting index (dialog)  Indices=PortIndex  OutputSizes=[1 1]
  Data Store Read : DataStoreRead  DataStoreName=SimCoreActuators  SampleTime=TimeStep
  Data Store Write : DataStoreWrite  DataStoreName=SimCoreActuators
  wires:
  Assignment/1 -> Data Store Write/1
  Data Store Read/1 -> Assignment/1
  Y/1 -> Assignment/2

== system OCT07_4_cs/STATE_Audi_A8_1/Position ==
  Y : Inport
  Assignment : Assignment  IndexMode=Zero-based  SampleTime=TimeStep  IndexOptions=Starting index (dialog)  Indices=PortIndex  OutputSizes=[1 1]
  Data Store Read : DataStoreRead  DataStoreName=SimCoreActuators  SampleTime=TimeStep
  Data Store Write : DataStoreWrite  DataStoreName=SimCoreActuators
  wires:
  Y/1 -> Assignment/2
  Data Store Read/1 -> Assignment/1
  Assignment/1 -> Data Store Write/1

== system OCT07_4_cs/STATE_Audi_A8_1/RPY ==
  Y : Inport
  Assignment : Assignment  IndexMode=Zero-based  SampleTime=TimeStep  IndexOptions=Starting index (dialog)  Indices=PortIndex  OutputSizes=[1 1]
  Data Store Read : DataStoreRead  DataStoreName=SimCoreActuators  SampleTime=TimeStep
  Data Store Write : DataStoreWrite  DataStoreName=SimCoreActuators
  wires:
  Assignment/1 -> Data Store Write/1
  Data Store Read/1 -> Assignment/1
  Y/1 -> Assignment/2

== system OCT07_4_cs/STATE_Audi_A8_1/Velocity ==
  Y : Inport
  Assignment : Assignment  IndexMode=Zero-based  SampleTime=TimeStep  IndexOptions=Starting index (dialog)  Indices=PortIndex  OutputSizes=[1 1]
  Data Store Read : DataStoreRead  DataStoreName=SimCoreActuators  SampleTime=TimeStep
  Data Store Write : DataStoreWrite  DataStoreName=SimCoreActuators
  wires:
  Assignment/1 -> Data Store Write/1
  Data Store Read/1 -> Assignment/1
  Y/1 -> Assignment/2

== system OCT07_4_cs/STATE_Audi_A8_1/velRPY ==
  Y : Inport
  Assignment : Assignment  IndexMode=Zero-based  SampleTime=TimeStep  IndexOptions=Starting index (dialog)  Indices=PortIndex  OutputSizes=[1 1]
  Data Store Read : DataStoreRead  DataStoreName=SimCoreActuators  SampleTime=TimeStep
  Data Store Write : DataStoreWrite  DataStoreName=SimCoreActuators
  wires:
  Assignment/1 -> Data Store Write/1
  Data Store Read/1 -> Assignment/1
  Y/1 -> Assignment/2

== system OCT07_4_cs/STATE_Toyota_Yaris_1/Acceleration ==
  Y : Inport
  Assignment : Assignment  IndexMode=Zero-based  SampleTime=TimeStep  IndexOptions=Starting index (dialog)  Indices=PortIndex  OutputSizes=[1 1]
  Data Store Read : DataStoreRead  DataStoreName=SimCoreActuators  SampleTime=TimeStep
  Data Store Write : DataStoreWrite  DataStoreName=SimCoreActuators
  wires:
  Assignment/1 -> Data Store Write/1
  Data Store Read/1 -> Assignment/1
  Y/1 -> Assignment/2

== system OCT07_4_cs/STATE_Toyota_Yaris_1/Position ==
  Y : Inport
  Assignment : Assignment  IndexMode=Zero-based  SampleTime=TimeStep  IndexOptions=Starting index (dialog)  Indices=PortIndex  OutputSizes=[1 1]
  Data Store Read : DataStoreRead  DataStoreName=SimCoreActuators  SampleTime=TimeStep
  Data Store Write : DataStoreWrite  DataStoreName=SimCoreActuators
  wires:
  Y/1 -> Assignment/2
  Data Store Read/1 -> Assignment/1
  Assignment/1 -> Data Store Write/1

== system OCT07_4_cs/STATE_Toyota_Yaris_1/RPY ==
  Y : Inport
  Assignment : Assignment  IndexMode=Zero-based  SampleTime=TimeStep  IndexOptions=Starting index (dialog)  Indices=PortIndex  OutputSizes=[1 1]
  Data Store Read : DataStoreRead  DataStoreName=SimCoreActuators  SampleTime=TimeStep
  Data Store Write : DataStoreWrite  DataStoreName=SimCoreActuators
  wires:
  Assignment/1 -> Data Store Write/1
  Data Store Read/1 -> Assignment/1
  Y/1 -> Assignment/2

== system OCT07_4_cs/STATE_Toyota_Yaris_1/Velocity ==
  Y : Inport
  Assignment : Assignment  IndexMode=Zero-based  SampleTime=TimeStep  IndexOptions=Starting index (dialog)  Indices=PortIndex  OutputSizes=[1 1]
  Data Store Read : DataStoreRead  DataStoreName=SimCoreActuators  SampleTime=TimeStep
  Data Store Write : DataStoreWrite  DataStoreName=SimCoreActuators
  wires:
  Assignment/1 -> Data Store Write/1
  Data Store Read/1 -> Assignment/1
  Y/1 -> Assignment/2

== system OCT07_4_cs/STATE_Toyota_Yaris_1/velRPY ==
  Y : Inport
  Assignment : Assignment  IndexMode=Zero-based  SampleTime=TimeStep  IndexOptions=Starting index (dialog)  Indices=PortIndex  OutputSizes=[1 1]
  Data Store Read : DataStoreRead  DataStoreName=SimCoreActuators  SampleTime=TimeStep
  Data Store Write : DataStoreWrite  DataStoreName=SimCoreActuators
  wires:
  Assignment/1 -> Data Store Write/1
  Data Store Read/1 -> Assignment/1
  Y/1 -> Assignment/2

== system OCT07_4_cs/Toyota_Yaris_1/Dynamics_Empty ==
  note: For state mode 'Dynamic' positions
      | are not taken into account, as they
      | are computed by integrating velocity.
      | Click annotation for Help.
  SteeringAngle : Inport
  "Acc " : Inport  Port=2
  V0 : Inport  Port=3
  Ground_{1..4} (4 alike) : Ground
  MuxState : Subsystem  Tag=MuxState  mask(Empty Dynamics State Block){positioningmode=on, TimeStep=1/20}
      mask prompts: positioningmode "Positioning Mode"; TimeStep "Auto Assigned: Time Step [s]"
      mask help:
      | Build the state of an actor based on user input.
      | The user can either use positioning mode or dynamics mode.
      | - When using positioning mode the position and orientation of the actor are set directly based on the input. Expected input is relative to the initial position and orientation of the actor. It's also possible to specify the velocity of the actor, though this input isn't used, only passed on.
      | - When using dynamics mode the position input is ignored. Expected input is velocity and orientation. The velocity is relative the current orientation of the actor, while orientation is relative to its initial orientation. The position of the actor is calculated based on the velocity and orientation given.
      settings: DeleteFcn=PreScanBlockDeleteFcn;
  Vehicle kinematics model : Subsystem
  degree2rad : Gain  Gain=pi/180
  State : Outport  Tag=StateOutport
  wires:
  Vehicle kinematics model/3(longitudinal position (x)) -> MuxState/1(x [m])
  Vehicle kinematics model/5(lateral position (y)) -> MuxState/2(y [m])
  Vehicle kinematics model/2(longitudinal vel (x dot)) -> MuxState/4(dx [m/s])
  Vehicle kinematics model/4(lateral vel (y dot)) -> MuxState/5(dy [m/s])
  Vehicle kinematics model/1(yaw angle (psi)) -> MuxState/9(Y [rad])
  "Acc "/1 -> Vehicle kinematics model/2(acceleration (a))
  V0/1 -> Vehicle kinematics model/3(initial vel (v0))
  SteeringAngle/1 -> degree2rad/1
  degree2rad/1 -> Vehicle kinematics model/1(steering angle (delta))
  MuxState/1(state) -> State/1
  Ground_1/1 -> MuxState/3(z [m])
  Ground_2/1 -> MuxState/6(dz [m/s])
  Ground_3/1 -> MuxState/7(R [rad])
  Ground_4/1 -> MuxState/8(P [rad])

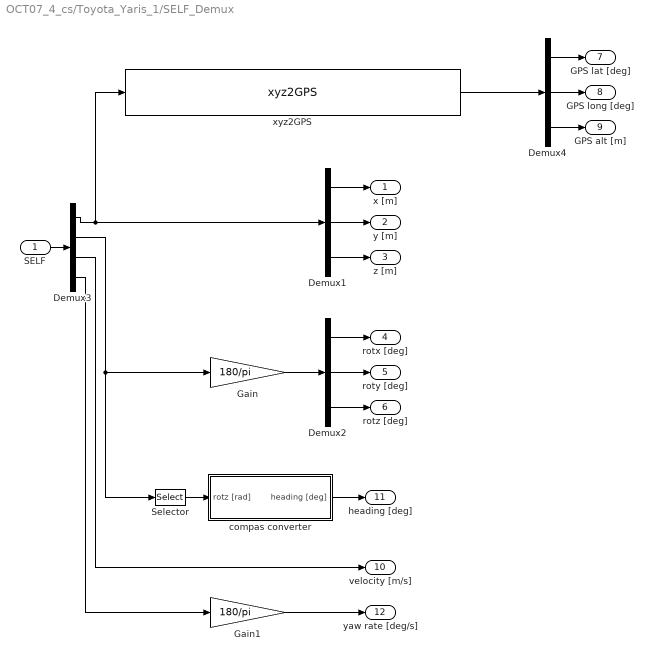
== system OCT07_4_cs/Toyota_Yaris_1/SELF_Demux ==
  SELF : Inport
  Demux1 : Demux  Outputs=3
  Demux2 : Demux  Outputs=3
  Demux3 : Demux  Outputs=[3 3 1 1]
  Demux4 : Demux  Outputs=3
  Gain : Gain  Gain=180/pi
  Gain1 : Gain  Gain=180/pi
  Selector : Selector  InputPortWidth=3  IndexOptions=Index vector (dialog)  Indices=[3]  OutputSizes=1
  compas converter : Subsystem
  xyz2GPS : PreScanUsefulBlocks/xyz2GPS  CoordinateCount=1  GPS_base=[0.000000 0.000000 0.000]
  x [m] : Outport
  y [m] : Outport  Port=2
  z [m] : Outport  Port=3
  rotx [deg] : Outport  Port=4
  roty [deg] : Outport  Port=5
  rotz [deg] : Outport  Port=6
  GPS lat [deg] : Outport  Port=7
  GPS long [deg] : Outport  Port=8
  GPS alt [m] : Outport  Port=9
  velocity [m/s] : Outport  Port=10
  heading [deg] : Outport  Port=11
  yaw rate [deg/s] : Outport  Port=12
  wires:
  Demux3/4 -> Gain1/1
  Gain1/1 -> yaw rate [deg/s]/1
  Demux3/3 -> velocity [m/s]/1
  compas converter/1(heading [deg]) -> heading [deg]/1
  xyz2GPS/1 -> Demux4/1
  Demux4/3 -> GPS alt [m]/1
  Demux4/2 -> GPS long [deg]/1
  Demux4/1 -> GPS lat [deg]/1
  Demux3/2 -> Gain/1, Selector/1
  Demux3/1 -> xyz2GPS/1, Demux1/1
  SELF/1 -> Demux3/1
  Demux2/3 -> rotz [deg]/1
  Demux2/2 -> roty [deg]/1
  Demux2/1 -> rotx [deg]/1
  Demux1/3 -> z [m]/1
  Demux1/2 -> y [m]/1
  Demux1/1 -> x [m]/1
  Gain/1 -> Demux2/1
  Selector/1 -> compas converter/1(rotz [rad])

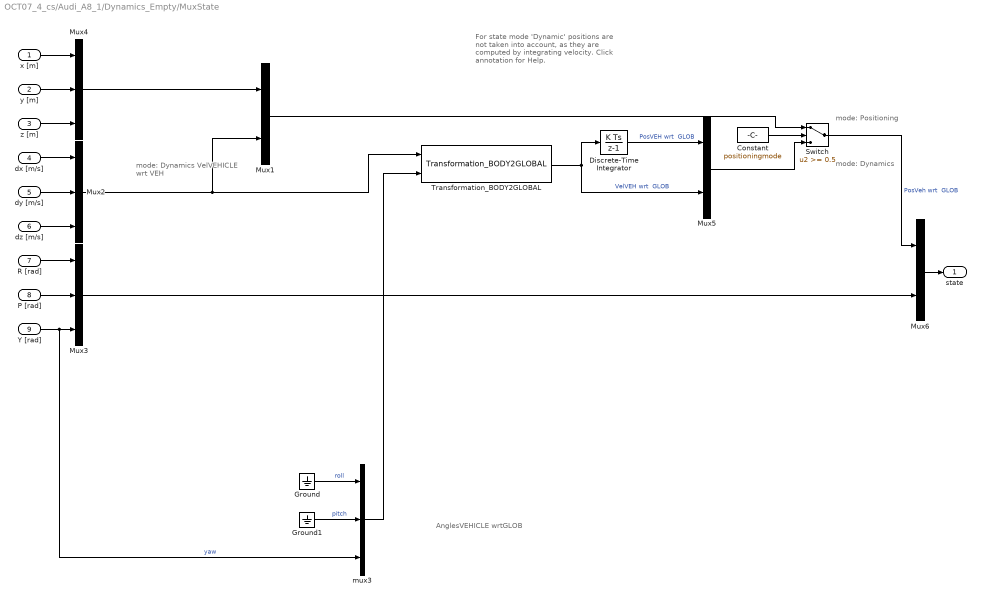
== system OCT07_4_cs/Audi_A8_1/Dynamics_Empty/MuxState ==
  note: mode: Dynamics
  note: mode: Positioning
  note: mode: Dynamics
      | VelVEHICLE
      | wrt VEH
  note: AnglesVEHICLE
      | wrtGLOB
  note: For state mode 'Dynamic' positions
      | are not taken into account, as they
      | are computed by integrating velocity.
      | Click annotation for Help.
  x [m] : Inport  SampleTime=TimeStep
  y [m] : Inport  Port=2  SampleTime=TimeStep
  z [m] : Inport  Port=3  SampleTime=TimeStep
  dx [m/s] : Inport  Port=4  SampleTime=TimeStep
  dy [m/s] : Inport  Port=5  SampleTime=TimeStep
  dz [m/s] : Inport  Port=6  SampleTime=TimeStep
  R [rad] : Inport  Port=7  SampleTime=TimeStep
  P [rad] : Inport  Port=8  SampleTime=TimeStep
  Y [rad] : Inport  Port=9  SampleTime=TimeStep
  Constant : Constant  DisableCoverage=on  Value=positioningmode
  Discrete-Time Integrator : DiscreteIntegrator  SampleTime=TimeStep  ICPrevOutput=DiscIntNeverNeededParam  ICPrevScaledInput=DiscIntNeverNeededParam
  Ground : Ground
  Ground1 : Ground
  Mux1 : Mux  Inputs=[3 3]
  Mux2 : Mux  Inputs=3
  Mux3 : Mux  Inputs=3
  Mux4 : Mux  Inputs=3
  Mux5 : Mux  Inputs=[3 3]
  Mux6 : Mux  Inputs=[6 3]
  Switch : Switch  Threshold=0.5
  Transformation_BODY2GLOBAL : PreScanSimulinkLibrary/Simple_Vehicle_Dynamics/Chassis/MuxDynState/Transformation_BODY2GLOBAL
  mux3 : Mux  Inputs=3
  state : Outport
  wires:
  Constant/1 -> Switch/2
  Mux6/1 -> state/1
  Mux4/1 -> Mux1/1
  Mux5/1 -> Switch/3
  Mux1/1 -> Switch/1
  Switch/1 -> Mux6/1  "PosVeh wrt  GLOB"
  P [rad]/1 -> Mux3/2
  R [rad]/1 -> Mux3/1
  dz [m/s]/1 -> Mux2/3
  dy [m/s]/1 -> Mux2/2
  dx [m/s]/1 -> Mux2/1
  z [m]/1 -> Mux4/3
  y [m]/1 -> Mux4/2
  x [m]/1 -> Mux4/1
  Ground1/1 -> mux3/2  "pitch"
  Y [rad]/1 -> mux3/3, Mux3/3  "yaw"
  Mux3/1 -> Mux6/2
  Transformation_BODY2GLOBAL/1 -> Discrete-Time Integrator/1, Mux5/2  "VelVEH wrt  GLOB"
  mux3/1 -> Transformation_BODY2GLOBAL/2
  Ground/1 -> mux3/1  "roll"
  Mux2/1 -> Mux1/2, Transformation_BODY2GLOBAL/1
  Discrete-Time Integrator/1 -> Mux5/1  "PosVEH wrt  GLOB"
